simulink model "Activity_9"  (R2019b)
settings: Solver=VariableStepAuto  StartTime=0.0  StopTime=0.1  RelTol=1e-3
libraries: dspsrcs4 x2, dspfdesign x1
settings Model: Creator=linesLK  LastModifiedBy=linesLK

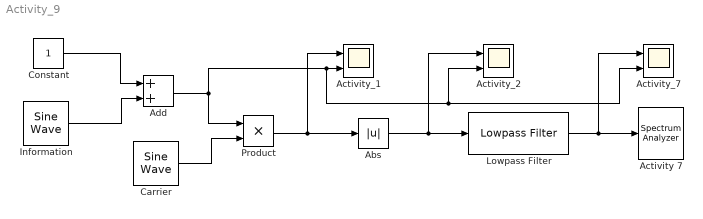
== system Activity_9 ==
  Abs : Abs
  Activity 7 : SpectrumAnalyzer
  Activity_1 : Scope  NumInputPorts=2
  Activity_2 : Scope  NumInputPorts=2
  Activity_7 : Scope  NumInputPorts=2
  Add : Sum
  Carrier : dspsrcs4/Sine Wave  Amplitude=1  Frequency=15000  Phase=pi/2  SampleMode=Discrete  OutComplex=Real  CompMethod=Trigonometric fcn  TableSize=Speed  SampleTime=1/120000  SamplesPerFrame=1  ResetState=Restart at time zero  OutputFrames=off  dataType=double  wordLen=16  udDataType=sfix(16)  fracBitsMode=Best precision  numFracBits=15  OutDataTypeStr=double  LastOutDataTypeStr=double
  Constant : Constant
  Information : dspsrcs4/Sine Wave  Amplitude=1  Frequency=1000  Phase=pi/2  SampleMode=Discrete  OutComplex=Real  CompMethod=Trigonometric fcn  TableSize=Speed  SampleTime=1/120000  SamplesPerFrame=1  ResetState=Restart at time zero  OutputFrames=off  dataType=double  wordLen=16  udDataType=sfix(16)  fracBitsMode=Best precision  numFracBits=15  OutDataTypeStr=double  LastOutDataTypeStr=double
  Lowpass Filter : dspfdesign/Lowpass Filter  FilterType=FIR  DesignForMinimumOrder=on  FilterOrder=100  PassbandFrequency=1e3  StopbandFrequency=15e3  PassbandRipple=0.1  StopbandAttenuation=80  InheritSampleRate=on  SampleRate=44100  SimulateUsing=Interpreted execution  roundingMode=Floor  coeffsDataTypeStr=fixdt(1,16)
  Product : Product
  wires:
  Lowpass Filter/1 -> Activity_7/1, Activity 7/1
  Abs/1 -> Activity_2/1, Lowpass Filter/1
  Carrier/1 -> Product/2
  Product/1 -> Activity_1/1, Abs/1
  Constant/1 -> Add/1
  Add/1 -> Product/1, Activity_2/2, Activity_7/2, Activity_1/2
  Information/1 -> Add/2
